simulink model "Caishidianlu_design_tu"  (R2016a)
settings: Solver=VariableStepAuto  SolverMode=SingleTasking  StartTime=0.0  StopTime=10  RelTol=1e-3
values from neighbouring files (symbols this model uses):
  C = [1 0 0]    [Caishidianlu_design.m]    (also in Daolibai_analysis_ControllAndObserv.m = [1 0 0 0]; Daolibai_analysis_stability.m = [1 0 0 0]; Daolibai_design_OSF.m = [1 0 0 0]; Daolibai_design_OSFandPIOF.m = [1 0 0 0])
  K = inv(P1)*V1    [Caishidianlu_design.m]    (also in Daolibai_design_OSF.m = acker(A1,B1,P1); Daolibai_design_OSFandPIOF.m = acker(A1,B1,P); Daolibai_design_SF.m = acker(A1,B1,P); Daolibai_design_SFandOF.m = acker(A,B,P))
settings Model: Creator=19017  LastModifiedBy=19017
settings DataIOCC: ReturnWorkspaceOutputs=on
settings DebuggingCC: SFUnexpectedBacktrackingDiag=error  SFNoUnconditionalDefaultTransitionDiag=error
settings SFSimCC: SimUseLocalCustomCode=on
settings RTWCC: RTWUseLocalCustomCode=on
settings GRTTargetCC: TargetLangStandard=C99 (ISO)
settings ConfigComp: CovMetricSettings=dwe  CovSaveCumulativeToWorkspaceVar=off  CovSaveSingleToWorkspaceVar=off  CovExternalEMLEnable=on

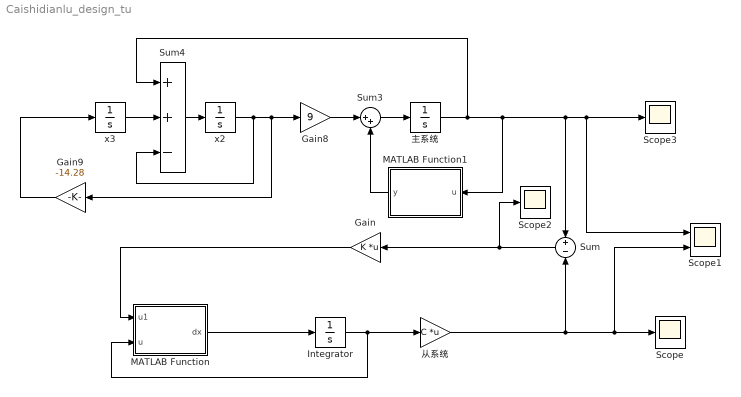
== system Caishidianlu_design_tu ==
  Gain : Gain  Gain=K  Multiplication=Matrix(K*u)
  Gain8 : Gain  Gain=9
  Gain9 : Gain  Gain=-14.28
  Integrator : Integrator  InitialCondition=[-0.5 0.5 2]
  MATLAB Function : MATLAB Function  TreatAsAtomicUnit=on
  MATLAB Function1 : MATLAB Function  TreatAsAtomicUnit=on
  Scope : Scope
  Scope1 : Scope  NumInputPorts=2
  Scope2 : Scope
  Scope3 : Scope
  Sum : Sum  Inputs=+|-
  Sum3 : Sum  Inputs=|++
  Sum4 : Sum  Inputs=++-
  x2 : Integrator  InitialCondition=0.1
  x3 : Integrator  InitialCondition=0.2
  主系统 : Integrator  InitialCondition=-0.1
  从系统 : Gain  Gain=C  Multiplication=Matrix(K*u)
  wires:
  MATLAB Function/1(dx) -> Integrator/1
  MATLAB Function1/1(y) -> Sum3/2
  Gain9/1 -> x3/1
  主系统/1 -> Scope1/1, Scope3/1, Sum/1, MATLAB Function1/1(u), Sum4/1
  x3/1 -> Sum4/2
  Gain8/1 -> Sum3/1
  Sum4/1 -> x2/1
  x2/1 -> Sum4/3, Gain9/1, Gain8/1
  Sum3/1 -> 主系统/1
  Integrator/1 -> MATLAB Function/2(u), 从系统/1
  从系统/1 -> Scope1/2, Scope/1, Sum/2
  Sum/1 -> Scope2/1, Gain/1
  Gain/1 -> MATLAB Function/1(u1)

== matlab function Caishidianlu_design_tu/MATLAB Function ==
  data: u1 input; u input; dx output
function dx = fcn(u1,u)
a=9;b=14.28;m0=-1/7;m1=2/7;c=1;
A=[ -a*m1,a,0;1,-2, 1;0, -b, 0];
H=[-a*(m0-m1);0;0];
C=[1,0,0];
D=[1,0,0];
W=1;
x1=u(1);
x2=u(2);
x3=u(3);
sigma=1/2*(abs(x1+c) - abs(x1-c));
dx1=-a*m1*x1+a*x2-a*(m0-m1)*sigma+u1(1);
dx2=x1-x2+x3+u1(2) ;
dx3=-b*x2+u1(3);
dx=[dx1;dx2;dx3];

== matlab function Caishidianlu_design_tu/MATLAB Function1 ==
  data: u input; y output
function y = fcn(u)
x1=u;
x1dao=-((2*9)/7)*x1+(((9*3)/7)/2)*(abs(x1+1)-abs(x1-1))
y=x1dao;
